simulink model "hexa_tilted_CAD_FxTESO_ANSFT"  (R2023a)
settings: Solver=ode4  StartTime=0.0  StopTime=60  FixedStep=0.01  RelTol=1e-3
model workspace (MAT data in the model file):
  hover_2m = [0 0 2 0 0 0 0 0 2 0 0 0 ... (36 elements, 6x6)]
  square = [0 0 2.5 0 0 0 0 0 2.5 0 0 0 ... (36 elements, 6x6)]
  tf : Simulink.Parameter (value not decoded)
  tray0 = [0 0 0 0 0 0 0 0 5 0 0 0 ... (36 elements, 6x6)]
  tray1 = [0 0 0 0 0 0 0 0 5 0 0 0 ... (36 elements, 6x6)]
  tray2 = [0 0 0 0 0 0 2 0 5 0 0 0 ... (36 elements, 6x6)]
  tray3 = [0 0 0 0 0 0 2 0 5 0 0 0 ... (36 elements, 6x6)]
  tray4 = [0 0 0 0 0 0 2 0 5 0.15 0 0 ... (36 elements, 6x6)]
  tray5 = [0 0 0 0 0 0 0 0 5 0.15 0 0 ... (36 elements, 6x6)]
  tray_yaw = [0 0 0 0 0 0 0 0 5 0 0 0 ... (36 elements, 6x6)]
undefined symbols (not defined in the file or in its folder): F, Light, MIL, smiData, X, Y, Z
libraries: sm_lib x229, nesl_utility x26, sharedtransform x2, robotcorelib x2, mspsensorlib x1, sensorinslib x1, simulink x1, aerolibwind2 x1, SignalEditorBlockLib x1
(part 2 of 6)

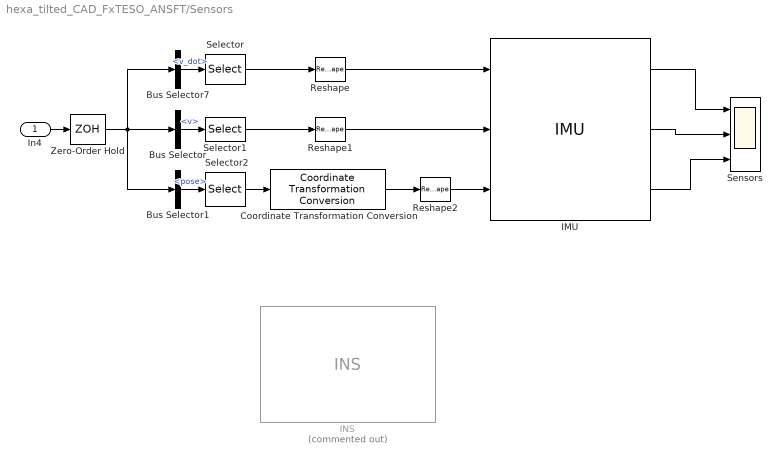
== system hexa_tilted_CAD_FxTESO_ANSFT/Sensors ==
  In4 : Inport
  Bus Selector : BusSelector  OutputSignals=v
  Bus Selector1 : BusSelector  OutputSignals=pose
  Bus Selector7 : BusSelector  OutputSignals=v_dot
  Coordinate Transformation Conversion : robotcorelib/Coordinate Transformation Conversion  InputRepresentation=Euler Angles  InputEulerSequence=ZYX  ShowTrVecInputPort=on  OutputRepresentation=Quaternion  OutputEulerSequence=ZYX  ShowTrVecOutputPort=on  SimulateUsing=Interpreted execution
      settings: LibrarySourceBlock=navlib/Utilities/Coordinate Transformation Conversion
  IMU : mspsensorlib/IMU  DispRefFrame=NED  Temperature=25  MagneticFieldNED=[ 27.5550, -2.4169, -16.0849 ]  MagneticFieldENU=[ -2.4169, 27.5550, 16.0849 ]  SeedDouble=67  SimulateUsing=Interpreted execution  AccelParamsMeasurementRange=Inf  AccelParamsResolution=0  AccelParamsConstantBias=[ 0, 0, 0 ]  AccelParamsAxesMisalignment=[ 100, 0, 0; 0, 100, 0; 0, 0, 100 ]  AccelParamsNoiseDensity=[ 0, 0, 0 ]  AccelParamsBiasInstability=[ 0, 0, 0 ]  AccelParamsRandomWalk=[ 0, 0, 0 ]  AccelParamsTemperatureBias=[ 0, 0, 0 ]  AccelParamsTemperatureScaleFactor=[ 0, 0, 0 ]  GyroParamsMeasurementRange=Inf  GyroParamsResolution=0  GyroParamsConstantBias=[ 0, 0, 0 ]  GyroParamsAxesMisalignment=[ 100, 0, 0; 0, 100, 0; 0, 0, 100 ]  GyroParamsAccelerationBias=[ 0, 0, 0 ]  GyroParamsNoiseDensity=[ 0, 0, 0 ]  GyroParamsBiasInstability=[ 0, 0, 0 ]  GyroParamsRandomWalk=[ 0, 0, 0 ]  GyroParamsTemperatureBias=[ 0, 0, 0 ]  GyroParamsTemperatureScaleFactor=[ 0, 0, 0 ]  MagParamsMeasurementRange=Inf  MagParamsResolution=0  MagParamsConstantBias=[ 0, 0, 0 ]  MagParamsAxesMisalignment=[ 100, 0, 0; 0, 100, 0; 0, 0, 100 ]  MagParamsNoiseDensity=[ 0, 0, 0 ]  MagParamsBiasInstability=[ 0, 0, 0 ]  MagParamsRandomWalk=[ 0, 0, 0 ]  MagParamsTemperatureBias=[ 0, 0, 0 ]  MagParamsTemperatureScaleFactor=[ 0, 0, 0 ]
  INS : sensorinslib/INS  Commented=on  MountingLocation=[0 0 0]  RollAccuracy=0.2  PitchAccuracy=0.2  YawAccuracy=1  PositionAccuracy=1  VelocityAccuracy=0.05  UseAccelAndAngVel=off  AccelerationAccuracy=0  AngularVelocityAccuracy=0  TimeInput=off  PositionErrorFactor=[0 0 0]  SeedDouble=67  SimulateUsing=Code generation
      settings: LibrarySourceBlock=drivingscenarioandsensors/INS
  Reshape : Reshape  OutputDimensionality=Row vector (2-D)
  Reshape1 : Reshape  OutputDimensionality=Row vector (2-D)
  Reshape2 : Reshape  OutputDimensionality=Row vector (2-D)
  Selector : Selector  InputPortWidth=6  IndexOptions=Index vector (dialog)  Indices=[1:3]  OutputSizes=1
  Selector1 : Selector  InputPortWidth=6  IndexOptions=Index vector (dialog)  Indices=[4:6]  OutputSizes=1
  Selector2 : Selector  InputPortWidth=6  IndexOptions=Index vector (dialog)  Indices=[6 5 4]  OutputSizes=1
  Sensors : Scope  NumInputPorts=3
  Zero-Order Hold : ZeroOrderHold  SampleTime=0.01
  wires:
  Bus Selector7/1 -> Selector/1  "<v_dot>"
  In4/1 -> Zero-Order Hold/1
  Selector/1 -> Reshape/1
  Bus Selector/1 -> Selector1/1  "<v>"
  Selector1/1 -> Reshape1/1
  Bus Selector1/1 -> Selector2/1  "<pose>"
  Selector2/1 -> Coordinate Transformation Conversion/1
  Coordinate Transformation Conversion/1 -> Reshape2/1
  IMU/2 -> Sensors/2
  IMU/1 -> Sensors/1
  IMU/3 -> Sensors/3
  Reshape1/1 -> IMU/2
  Reshape/1 -> IMU/1
  Reshape2/1 -> IMU/3
  Zero-Order Hold/1 -> Bus Selector7/1, Bus Selector1/1, Bus Selector/1

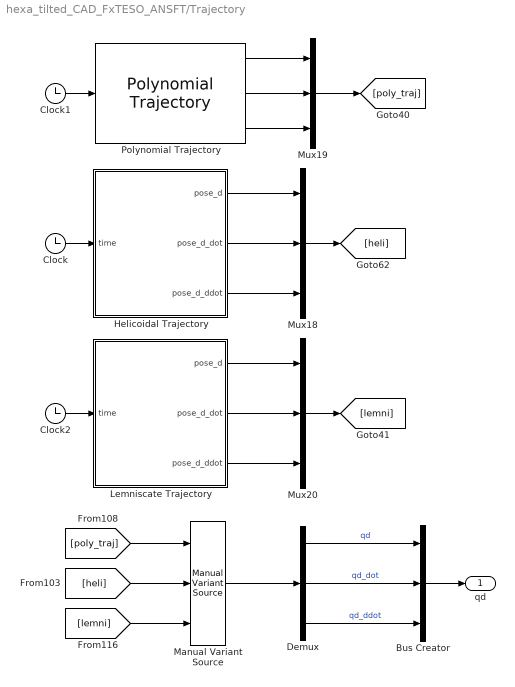
== system hexa_tilted_CAD_FxTESO_ANSFT/Trajectory ==
  Bus Creator : BusCreator  Inputs=3
  Clock : Clock
  Clock1 : Clock
  Clock2 : Clock
  Demux : Demux  Outputs=3
  Helicoidal Trajectory : MATLAB Function  TreatAsAtomicUnit=on
  Lemniscate Trajectory : MATLAB Function  TreatAsAtomicUnit=on
  Manual Variant Source : simulink/Signal Routing/Manual Variant Source  NumChoices=3  LabelModeActiveChoice=V_1
  Mux18 : Mux  Inputs=3
  Mux19 : Mux  Inputs=3
  Mux20 : Mux  Inputs=3
  Polynomial Trajectory : robotcorelib/Polynomial Trajectory  WaypointSource=Internal  Waypoints=zeros(6, 6)  TimePoints=[ 0, 12, 24, 36, 48, tf ]  TimeInterval=[ 1, 4 ]  Method=Cubic Polynomial  ParameterSource=Internal  VelocityBoundaryCondition=zeros( 6, 6 )  AccelerationBoundaryCondition=zeros( 2, 5 )  SimulateUsing=Interpreted execution
  qd : Outport
  wires:
  Manual Variant Source/1 -> Demux/1
  Lemniscate Trajectory/2(pose_d_dot) -> Mux20/2
  [poly_traj] -> Manual Variant Source/1
  Polynomial Trajectory/3 -> Mux19/3
  Helicoidal Trajectory/1(pose_d) -> Mux18/1
  Clock1/1 -> Polynomial Trajectory/1
  Mux18/1 -> [heli]
  Lemniscate Trajectory/3(pose_d_ddot) -> Mux20/3
  Polynomial Trajectory/2 -> Mux19/2
  Demux/2 -> Bus Creator/2  "qd_dot"
  Clock2/1 -> Lemniscate Trajectory/1(time)
  Helicoidal Trajectory/3(pose_d_ddot) -> Mux18/3
  Demux/1 -> Bus Creator/1  "qd"
  Mux19/1 -> [poly_traj]
  Mux20/1 -> [lemni]
  Lemniscate Trajectory/1(pose_d) -> Mux20/1
  Helicoidal Trajectory/2(pose_d_dot) -> Mux18/2
  Clock/1 -> Helicoidal Trajectory/1(time)
  Demux/3 -> Bus Creator/3  "qd_ddot"
  [heli] -> Manual Variant Source/2
  [lemni] -> Manual Variant Source/3
  Bus Creator/1 -> qd/1
  Polynomial Trajectory/1 -> Mux19/1

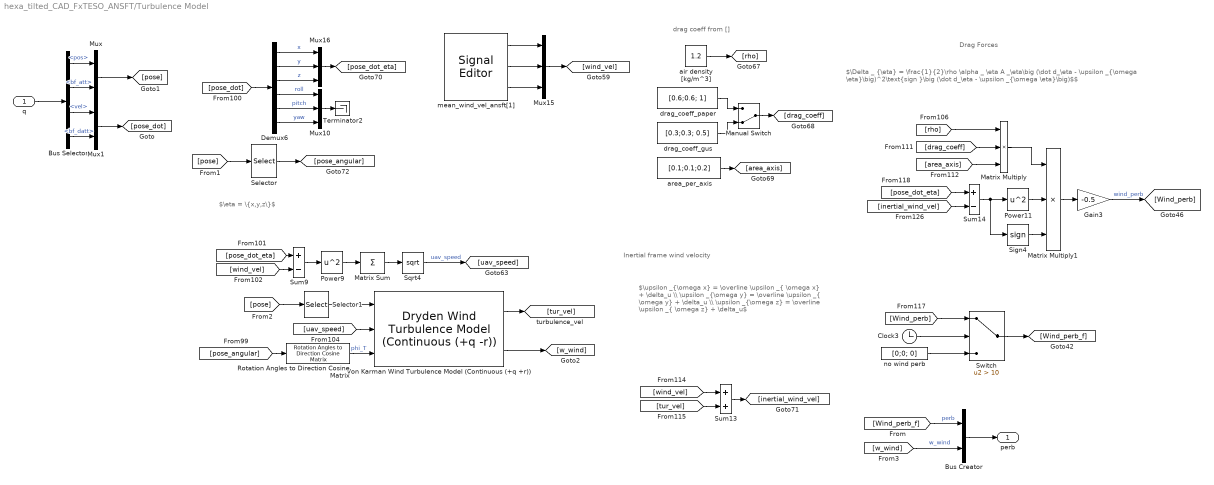
== system hexa_tilted_CAD_FxTESO_ANSFT/Turbulence Model ==
  note: $\Delta _ {\eta} = \frac{1}{2}\rho \alpha _ \eta A _\eta\big (\dot d_\eta - \upsilon _{\omega \eta}\big)^2\text{sign }\big (\dot d_\eta - \upsilon _{\omega \eta}\big)$$
  note: drag coeff from []
  note: $\upsilon _{\omega x} = \overline \upsilon _{ \omega x} + \delta_u \\ \upsilon _{\omega y} = \overline \upsilon _{ \omega y} + \delta_u \\ \upsilon _{\omega z} = \overline \upsilon _{ \omega z} + \delta_u$
  note: $\eta = \{x,y,z\}$
  note: Drag Forces
  note: Inertial frame wind velocity
  q : Inport
  Bus Creator : BusCreator  Inputs=2
  Bus Selector : BusSelector  OutputSignals=pos,bf_att,vel,bf_datt
  Clock3 : Clock
  Demux6 : Demux  Outputs=6
  Gain3 : Gain  Gain=-0.5
  Manual Switch : ManualSwitch  CurrentSetting=0
  Matrix Sum : Sum  Inputs=+
  Matrix Multiply : Product  Inputs=3
  Matrix Multiply1 : Product  Inputs=3
  Mux : Mux  Inputs=2
  Mux1 : Mux  Inputs=2
  Mux10 : Mux  Inputs=3
  Mux15 : Mux  Inputs=3
  Mux16 : Mux  Inputs=3
  Power11 : Math  Operator=square
  Power9 : Math  Operator=square
  Rotation Angles to Direction Cosine Matrix : sharedtransform/Rotation Angles to Direction Cosine Matrix  rotationOrder=ZYX  aMode=aMode
  Selector : Selector  InputPortWidth=6  IndexOptions=Index vector (dialog)  Indices=[4:6]  OutputSizes=1
  Selector1 : Selector  InputPortWidth=6  IndexOptions=Index vector (dialog)  Indices=[3]  OutputSizes=1
  Sign4 : Signum
  Sqrt4 : Sqrt
  Sum13 : Sum
  Sum14 : Sum  Inputs=+-
  Sum9 : Sum  Inputs=+-
  Switch : Switch  Criteria=u2 > Threshold  Threshold=10  SaturateOnIntegerOverflow=off  InputSameDT=off
  Terminator2 : Terminator
  Von Karman Wind Turbulence Model (Continuous (+q +r)) : aerolibwind2/Dryden Wind Turbulence Model  (Continuous (+q -r))  units=Metric (MKS)  spec=MIL-F-8785C  model=Continuous Von Karman (+q -r)  W20=15  Wdeg=0  TurbProb=10^-2 - Light  L_high=762  Wingspan=10  ts=0.1  Seed=[23341 23342 23343 23344]  T_on=on
      settings: LibrarySourceBlock=|
      | aerolibwind2/Von Karman Wind Turbulence Model
      | (Continuous (+q +r))
  air density [kg/m^3] : Constant  Value=1.2
  area_per_axis : Constant  Value=[0.1;0.1;0.2]
  drag_coeff_gus : Constant  Value=[0.3;0.3; 0.5]
  drag_coeff_paper : Constant  Value=[0.6;0.6; 1]
  mean_wind_vel_ansft[1] : SignalEditorBlockLib/Signal Editor  FileName=mean_wind_vel_ansft.mat  ActiveScenario=Velocidades_medias_del_viento  ActiveSignal=wean_wind_vel_x  IsBus=off  OutputBusObjectStr=Bus: BusObject  SampleTime=0  Interpolate=off  ZeroCross=off  OutputAfterFinalValue=Setting to zero  Unit=inherit  PreserveSignalName=on  ApplySigPropsToAllScenarios=on
  no wind perb : Constant  Value=[0;0; 0]
  perb : Outport
  wires:
  mean_wind_vel_ansft[1]/2 -> Mux15/2
  Demux6/1 -> Mux16/1  "x"
  mean_wind_vel_ansft[1]/1 -> Mux15/1
  [rho] -> Matrix Multiply/1
  Demux6/3 -> Mux16/3  "z"
  Manual Switch/1 -> [drag_coeff]
  Power11/1 -> Matrix Multiply1/2
  Von Karman Wind Turbulence Model (Continuous (+q +r))/1 -> [tur_vel]
  Rotation Angles to Direction Cosine Matrix/1 -> Von Karman Wind Turbulence Model (Continuous (+q +r))/3  "phi_T"
  drag_coeff_paper/1 -> Manual Switch/1
  Matrix Sum/1 -> Sqrt4/1
  Gain3/1 -> [Wind_perb]  "wind_perb"
  Matrix Multiply/1 -> Matrix Multiply1/1
  Selector/1 -> [pose_angular]
  Sum9/1 -> Power9/1
  no wind perb/1 -> Switch/3
  Mux16/1 -> [pose_dot_eta]
  Clock3/1 -> Switch/2
  Sum14/1 -> Sign4/1, Power11/1
  [area_axis] -> Matrix Multiply/3
  Von Karman Wind Turbulence Model (Continuous (+q +r))/2 -> [w_wind]
  [uav_speed] -> Von Karman Wind Turbulence Model (Continuous (+q +r))/2
  Demux6/4 -> Mux10/1  "roll"
  Mux15/1 -> [wind_vel]
  [drag_coeff] -> Matrix Multiply/2
  air density [kg/m^3]/1 -> [rho]
  Mux10/1 -> Terminator2/1
  area_per_axis/1 -> [area_axis]
  [pose_angular] -> Rotation Angles to Direction Cosine Matrix/1
  drag_coeff_gus/1 -> Manual Switch/2
  Sum13/1 -> [inertial_wind_vel]
  Switch/1 -> [Wind_perb_f]
  [pose_dot_eta] -> Sum9/1
  Demux6/5 -> Mux10/2  "pitch"
  [tur_vel] -> Sum13/2
  Selector1/1 -> Von Karman Wind Turbulence Model (Continuous (+q +r))/1
  [pose_dot_eta] -> Sum14/1
  [wind_vel] -> Sum9/2
  [Wind_perb] -> Switch/1
  [wind_vel] -> Sum13/1
  Sqrt4/1 -> [uav_speed]  "uav_speed"
  Demux6/6 -> Mux10/3  "yaw"
  Sign4/1 -> Matrix Multiply1/3
  Demux6/2 -> Mux16/2  "y"
  mean_wind_vel_ansft[1]/3 -> Mux15/3
  Power9/1 -> Matrix Sum/1
  Matrix Multiply1/1 -> Gain3/1
  [pose_dot] -> Demux6/1
  [inertial_wind_vel] -> Sum14/2
  Bus Creator/1 -> perb/1
  [Wind_perb_f] -> Bus Creator/1  "perb"
  q/1 -> Bus Selector/1
  [pose] -> Selector/1
  [pose] -> Selector1/1
  [w_wind] -> Bus Creator/2  "w_wind"
  Bus Selector/2 -> Mux/2  "<bf_att>"
  Bus Selector/1 -> Mux/1  "<pos>"
  Mux/1 -> [pose]
  Bus Selector/3 -> Mux1/1  "<vel>"
  Bus Selector/4 -> Mux1/2  "<bf_datt>"
  Mux1/1 -> [pose_dot]

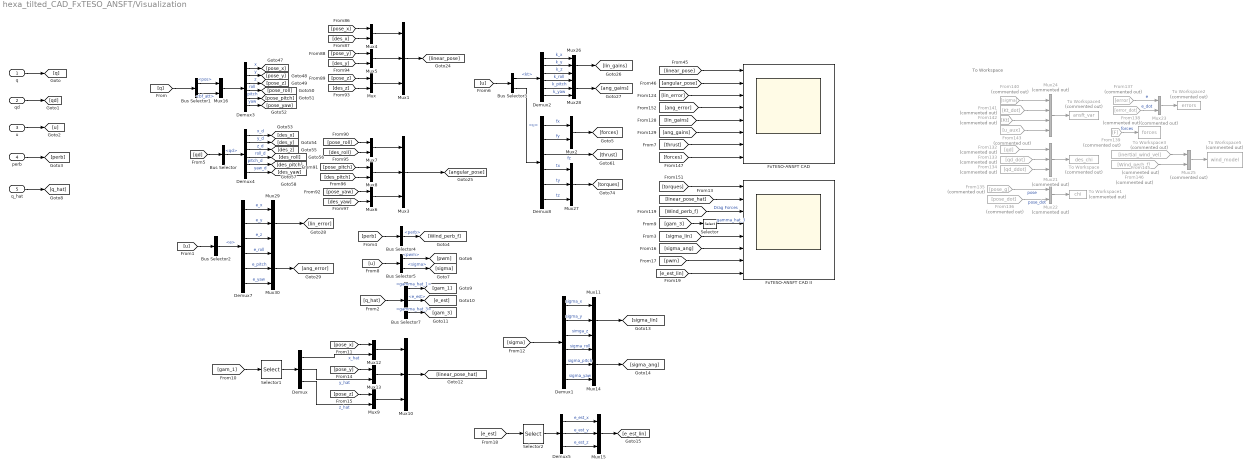
== system hexa_tilted_CAD_FxTESO_ANSFT/Visualization ==
  note: To Workspace
  q : Inport
  qd : Inport  Port=2
  u : Inport  Port=3
  perb : Inport  Port=4
  q_hat : Inport  Port=5
  Bus Selector : BusSelector  OutputSignals=qd
  Bus Selector1 : BusSelector  OutputSignals=pos,bf_att
  Bus Selector2 : BusSelector  OutputSignals=e
  Bus Selector3 : BusSelector  OutputSignals=kt,u
  Bus Selector4 : BusSelector  OutputSignals=perb
  Bus Selector5 : BusSelector  OutputSignals=pwm,sigma
  Bus Selector7 : BusSelector  OutputSignals=gamma_hat_1,e_est,gamma_hat_3
  Demux : Demux  Outputs=3
  Demux{1..4,7..8} (6 alike) : Demux  Outputs=6
  Demux5 : Demux  Outputs=3
  From132 : From  Commented=on  GotoTag=qd
  From133 : From  Commented=on  GotoTag=qd_dot
  From134 : From  Commented=on  GotoTag=qd_ddot
  From135 : From  Commented=on  GotoTag=pose_g
  From136 : From  Commented=on  GotoTag=pose_dot
  From137 : From  Commented=on  GotoTag=error
  From138 : From  Commented=on  GotoTag=error_dot
  From139 : From  Commented=on  GotoTag=F
  From140 : From  Commented=on  GotoTag=sigma
  From141 : From  Commented=on  GotoTag=Kt_dot
  From142 : From  Commented=on  GotoTag=Kt
  From143 : From  Commented=on  GotoTag=u_aux
  From145 : From  Commented=on  GotoTag=inertial_wind_vel
  From146 : From  Commented=on  GotoTag=Wind_perb_f
  FxTESO-ANSFT CAD : Scope  NumInputPorts=8
  FxTESO-ANSFT CAD II : Scope  NumInputPorts=8
  Mux{,2,4..9,12..13,16} (11 alike) : Mux  Inputs=2
  Mux{1,3,10..11,14..15,26..30} (11 alike) : Mux  Inputs=3
  Mux21 : Mux  Commented=on  Inputs=3
  Mux22 : Mux  Commented=on  Inputs=2
  Mux23 : Mux  Commented=on  Inputs=2
  Mux24 : Mux  Commented=on
  Mux25 : Mux  Commented=on  Inputs=2
  Selector : Selector  InputPortWidth=6  IndexOptions=Index vector (dialog)  Indices=[1:3]  OutputSizes=1
  Selector1 : Selector  InputPortWidth=6  IndexOptions=Index vector (dialog)  Indices=[1:3]  OutputSizes=1
  Selector2 : Selector  InputPortWidth=6  IndexOptions=Index vector (dialog)  Indices=[1:3]  OutputSizes=1
  To Workspace : ToWorkspace  Commented=on  VariableName=des_chi  SaveFormat=Structure With Time  SampleTime=-1
  To Workspace1 : ToWorkspace  Commented=on  VariableName=chi  SaveFormat=Structure With Time  SampleTime=-1
  To Workspace2 : ToWorkspace  Commented=on  VariableName=errors  SaveFormat=Structure With Time  SampleTime=-1
  To Workspace3 : ToWorkspace  Commented=on  VariableName=forces  SaveFormat=Structure With Time  SampleTime=-1
  To Workspace4 : ToWorkspace  Commented=on  VariableName=ansft_var  SaveFormat=Structure With Time  SampleTime=-1
  To Workspace5 : ToWorkspace  Commented=on  VariableName=wind_model  SaveFormat=Structure With Time  SampleTime=-1
  wires:
  Demux2/2 -> Mux26/2  "k_y"
  From137/1 -> Mux23/1  "e"
  Mux6/1 -> Mux3/3
  Mux25/1 -> To Workspace5/1
  Mux26/1 -> [lin_gains]
  Demux3/4 -> [pose_roll]  "roll"
  From145/1 -> Mux25/1
  Demux8/3 -> [thrust]  "fz"
  Mux2/1 -> [forces]
  From143/1 -> Mux24/4
  From132/1 -> Mux21/1
  Demux7/5 -> Mux30/2  "e_pitch"
  From142/1 -> Mux24/3
  From140/1 -> Mux24/1
  From135/1 -> Mux22/1  "pose"
  Demux7/6 -> Mux30/3  "e_yaw"
  From136/1 -> Mux22/2  "pose_dot"
  Mux3/1 -> [angular_pose]
  Mux5/1 -> Mux1/2
  [pose_x] -> Mux4/1
  [pose_z] -> Mux/1
  Mux21/1 -> To Workspace/1
  Bus Selector7/2 -> [e_est]  "<e_est>"
  [Wind_perb_f] -> FxTESO-ANSFT CAD II/3  "Drag Forces"
  Demux8/4 -> Mux27/1  "tx"
  Mux/1 -> Mux1/3
  [q_hat] -> Bus Selector7/1
  Demux3/1 -> [pose_x]  "x"
  Bus Selector4/1 -> [Wind_perb_f]  "<perb>"
  Mux4/1 -> Mux1/1
  Demux7/3 -> Mux29/3  "e_z"
  From141/1 -> Mux24/2
  [des_pitch] -> Mux8/2
  [perb] -> Bus Selector4/1
  Demux4/5 -> [des_pitch]  "pitch_d"
  [gam_3] -> Selector/1
  Mux7/1 -> Mux3/1
  Demux4/2 -> [des_y]  "y_d"
  Demux8/2 -> Mux2/2  "fy"
  Demux2/3 -> Mux26/3  "k_z"
  [qd] -> Bus Selector/1
  Mux28/1 -> [ang_gains]
  [u] -> Bus Selector2/1
  [u] -> Bus Selector3/1
  Mux1/1 -> [linear_pose]
  Mux24/1 -> To Workspace4/1
  Demux3/3 -> [pose_z]  "z"
  Mux8/1 -> Mux3/2
  From133/1 -> Mux21/2
  Selector/1 -> FxTESO-ANSFT CAD II/4  "gamma_hat_3"
  [u] -> Bus Selector5/1
  Mux22/1 -> To Workspace1/1
  Bus Selector3/2 -> Demux8/1  "<u>"
  Demux2/1 -> Mux26/1  "k_x"
  Mux30/1 -> [ang_error]
  [des_y] -> Mux5/2
  Demux2/4 -> Mux28/1  "k_roll"
  From139/1 -> To Workspace3/1  "forces"
  Bus Selector7/1 -> [gam_1]  "<gamma_hat_1>"
  [des_yaw] -> Mux6/2
  Mux27/1 -> [torques]
  Demux8/5 -> Mux27/2  "ty"
  From146/1 -> Mux25/2
  Bus Selector5/2 -> [sigma]  "<sigma>"
  Demux4/3 -> [des_z]  "z_d"
  Demux2/6 -> Mux28/3  "k_yaw"
  From138/1 -> Mux23/2  "e_dot"
  Demux3/6 -> [pose_yaw]  "yaw"
  Demux8/6 -> Mux27/3  "tz"
  Demux3/5 -> [pose_pitch]  "pitch"
  Demux4/1 -> [des_x]  "x_d"
  [pose_y] -> Mux5/1
  [des_x] -> Mux4/2
  Demux7/1 -> Mux29/1  "e_x"
  [linear_pose] -> FxTESO-ANSFT CAD/1
  Demux8/1 -> Mux2/1  "fx"
  [pose_pitch] -> Mux8/1
  Mux29/1 -> [lin_error]
  [pose_yaw] -> Mux6/1
  [q] -> Bus Selector1/1
  [des_roll] -> Mux7/2
  Demux2/5 -> Mux28/2  "k_pitch"
  [pose_roll] -> Mux7/1
  Mux23/1 -> To Workspace2/1
  Demux4/4 -> [des_roll]  "roll_d"
  Demux3/2 -> [pose_y]  "y"
  Demux4/6 -> [des_yaw]  "yaw_d"
  Bus Selector3/1 -> Demux2/1  "<kt>"
  Bus Selector2/1 -> Demux7/1  "<e>"
  Demux7/2 -> Mux29/2  "e_y"
  Demux7/4 -> Mux30/1  "e_roll"
  Bus Selector7/3 -> [gam_3]  "<gamma_hat_3>"
  [des_z] -> Mux/2
  Bus Selector/1 -> Demux4/1  "<qd>"
  [angular_pose] -> FxTESO-ANSFT CAD/2
  Bus Selector5/1 -> [pwm]  "<pwm>"
  From134/1 -> Mux21/3
  q/1 -> [q]
  qd/1 -> [qd]
  u/1 -> [u]
  perb/1 -> [perb]
  q_hat/1 -> [q_hat]
  [lin_error] -> FxTESO-ANSFT CAD/3
  [ang_error] -> FxTESO-ANSFT CAD/4
  [lin_gains] -> FxTESO-ANSFT CAD/5
  [ang_gains] -> FxTESO-ANSFT CAD/6
  [thrust] -> FxTESO-ANSFT CAD/7
  [forces] -> FxTESO-ANSFT CAD/8
  [torques] -> FxTESO-ANSFT CAD II/1
  Demux/1 -> Mux12/2  "x_hat"
  Mux9/1 -> Mux10/3
  [pose_z] -> Mux9/1
  Mux10/1 -> [linear_pose_hat]
  Mux12/1 -> Mux10/1
  Demux/3 -> Mux9/2  "z_hat"
  Demux/2 -> Mux13/2  "y_hat"
  [pose_y] -> Mux13/1
  Mux13/1 -> Mux10/2
  [pose_x] -> Mux12/1
  [gam_1] -> Selector1/1
  Selector1/1 -> Demux/1
  [linear_pose_hat] -> FxTESO-ANSFT CAD II/2
  Demux1/3 -> Mux11/3  "simga_z"
  Demux1/4 -> Mux14/1  "sigma_roll"
  Demux1/6 -> Mux14/3  "sigma_yaw"
  Demux1/2 -> Mux11/2  "sigma_y"
  [sigma] -> Demux1/1
  Mux11/1 -> [sigma_lin]
  Demux1/1 -> Mux11/1  "sigma_x"
  Demux1/5 -> Mux14/2  "sigma_pitch"
  Mux14/1 -> [sigma_ang]
  [sigma_lin] -> FxTESO-ANSFT CAD II/5
  [sigma_ang] -> FxTESO-ANSFT CAD II/6
  [pwm] -> FxTESO-ANSFT CAD II/7
  [e_est] -> Selector2/1
  Selector2/1 -> Demux5/1
  Demux5/3 -> Mux15/3  "e_est_z"
  Demux5/2 -> Mux15/2  "e_est_y"
  Demux5/1 -> Mux15/1  "e_est_x"
  Mux15/1 -> [e_est_lin]
  [e_est_lin] -> FxTESO-ANSFT CAD II/8
  Bus Selector1/1 -> Mux16/1  "<pos>"
  Bus Selector1/2 -> Mux16/2  "<bf_att>"
  Mux16/1 -> Demux3/1
